simulink library "sm_metronome_lib"  (R2026a)
settings: Solver=VariableStepAuto
undefined symbols (not defined in the file): metronome, X, Y, Z
libraries: sm_lib x11, nesl_utility x3
Description:
  | Copyright 2022-2026 The MathWorks, Inc.
settings Model: Creator=smiller  LastModifiedBy=smiller

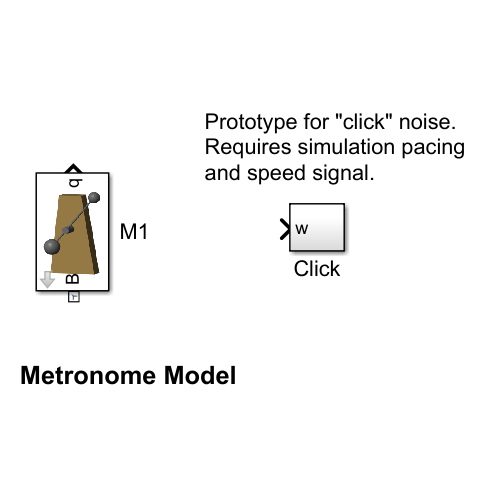
[thumbnail: Simulink's stored preview of the top-level diagram]
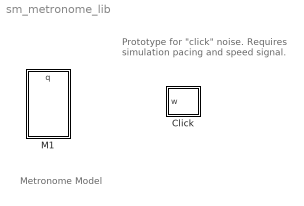
== system sm_metronome_lib ==
  note: Prototype for "click" noise. Requires simulation pacing and speed signal.
  note: Metronome Model
  Click : Subsystem
  M1 : Subsystem  mask(Metronome){pivot_h=metronome.pivot_h, len=metronome.stem_length, upper_len=metronome.stem_upper, upper_len_var=metronome.stem_upper_var, upper_m=metronome.upper_mass, lower_m=metronome.lower_mass, b_pivot=metronome.b_pivot, esc_torque=metronome.esc_torque, t0_ang=metronome.initial_angle(1), t0_vel=metronome.initial_speed(1)}
      mask prompts: pivot_h "Pivot Height (m)"; len "Stem Length (m)"; upper_len "Upper Stem/Length (0-1)"; upper_len_var "Variation in Upper Mass Location (m)"; upper_m "Mass Upper (m)"; lower_m "Mass Lower (m)"; b_pivot "Pivot Viscous Friction (N*m/(deg/s^2))"; esc_torque "Escapement Excitation Torque (N*m)"; t0_ang "Initial Angle (deg)"; t0_vel "Initial Speed (deg/s)"
      mask help: Models a metronome. The pendulum can swing back and forth. Contains abstract model of the energy imparted to the pendulum by the escapement mechanism.
      mask Display: image('sm_metronome_sync_metronome.png');

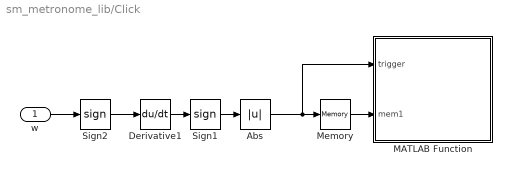
== system sm_metronome_lib/Click ==
  w : Inport
  Abs : Abs  SaturateOnIntegerOverflow=off
  Derivative1 : Derivative
  MATLAB Function : MATLAB Function  TreatAsAtomicUnit=on
  Memory : Memory  InheritSampleTime=on
  Sign1 : Signum
  Sign2 : Signum
  wires:
  Sign2/1 -> Derivative1/1
  Memory/1 -> MATLAB Function/2(mem1)
  w/1 -> Sign2/1
  Sign1/1 -> Abs/1
  Abs/1 -> Memory/1, MATLAB Function/1(trigger)
  Derivative1/1 -> Sign1/1

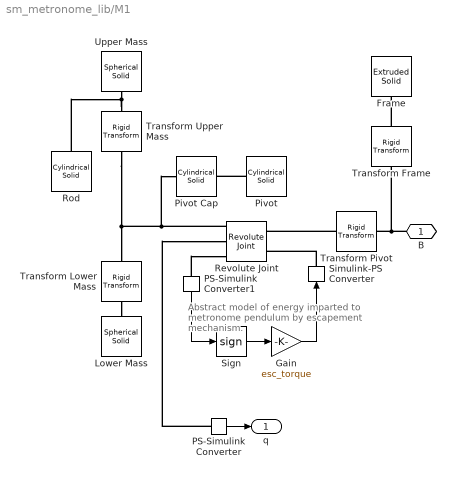
== system sm_metronome_lib/M1 ==
  note: Abstract model of energy imparted
      | to metronome pendulum
      | by escapement mechanism.
  Frame : sm_lib/Body Elements/Extruded Solid  ExtrusionType=General  PolygonNumSides=3  PolygonOuterRadius=1  PolygonOuterRadiusUnits=m  ExportEntireGeometry=off  ExtrusionCrossSection=[4 0; 2 14; -2 14; -4 0]/100  ExtrusionCrossSectionUnits=m  ExportConvexHullGeometry=off  ExtrusionLength=0.02  ExtrusionLengthUnits=m  InertiaType=CalculateFromGeometry  BasedOnType=Mass  Density=1000  DensityUnits=kg/m^3  Mass=0  MassUnits=kg  CenterOfMass=[0 0 0]  CenterOfMassUnits=m  MomentsOfInertia=[1 1 1]  MomentsOfInertiaUnits=kg*m^2  ProductsOfInertia=[0 0 0]  ProductsOfInertiaUnits=kg*m^2  GraphicType=FromGeometry  MarkerShape=Sphere  MarkerSize=10  GraphicVisPropType=SimpleVisualProperties  GraphicDiffuseColor=[0.7372549 0.6039216 0.3372549]  GraphicOpacity=1.0  GraphicSpecularColor=[0.5 0.5 0.5 1.0]  GraphicAmbientColor=[0.15 0.15 0.15 1.0]  GraphicEmissiveColor=[0.0 0.0 0.0 1.0]  GraphicShininess=75  DoExposeReferenceFrame=on  SerializedFrames=<Frames/>
  Gain : Gain  Gain=esc_torque
  Lower Mass : sm_lib/Body Elements/Spherical Solid  SphereRadius=0.014  SphereRadiusUnits=m  ExportEntireGeometry=off  InertiaType=CalculateFromGeometry  BasedOnType=Mass  Density=7600  DensityUnits=kg/m^3  Mass=lower_m  MassUnits=kg  CenterOfMass=[0 0 0]  CenterOfMassUnits=m  MomentsOfInertia=[1 1 1]  MomentsOfInertiaUnits=kg*m^2  ProductsOfInertia=[0 0 0]  ProductsOfInertiaUnits=kg*m^2  GraphicType=FromGeometry  MarkerShape=Sphere  MarkerSize=10  GraphicVisPropType=SimpleVisualProperties  GraphicDiffuseColor=[0.5 0.5 0.5]  GraphicOpacity=1.0  GraphicSpecularColor=[0.5 0.5 0.5 1.0]  GraphicAmbientColor=[0.15 0.15 0.15 1.0]  GraphicEmissiveColor=[0.0 0.0 0.0 1.0]  GraphicShininess=75  DoExposeReferenceFrame=on  SerializedFrames=<Frames/>
  PS-Simulink Converter : nesl_utility/PS-Simulink Converter  PhysicalDomain=network_engine_domain  SubClassName=ps_output  LeftPortType=input  RightPortType=output  PseudoPeriodic=off  Frequencies=[]  VectorFormat=1-D array  Unit=inherit  AffineConversion=off
  PS-Simulink Converter1 : nesl_utility/PS-Simulink Converter  PhysicalDomain=network_engine_domain  SubClassName=ps_output  LeftPortType=input  RightPortType=output  PseudoPeriodic=off  Frequencies=[]  VectorFormat=1-D array  Unit=inherit  AffineConversion=off
  Pivot : sm_lib/Body Elements/Cylindrical Solid  CylinderRadius=len/20  CylinderRadiusUnits=m  CylinderLength=0.03  CylinderLengthUnits=m  ExportEntireGeometry=off  InertiaType=CalculateFromGeometry  BasedOnType=Mass  Density=0  DensityUnits=kg/m^3  Mass=0  MassUnits=kg  CenterOfMass=[0 0 0]  CenterOfMassUnits=m  MomentsOfInertia=[1 1 1]  MomentsOfInertiaUnits=kg*m^2  ProductsOfInertia=[0 0 0]  ProductsOfInertiaUnits=kg*m^2  GraphicType=FromGeometry  MarkerShape=Sphere  MarkerSize=10  GraphicVisPropType=SimpleVisualProperties  GraphicDiffuseColor=[0.5 0.5 0.5]  GraphicOpacity=1.0  GraphicSpecularColor=[0.5 0.5 0.5 1.0]  GraphicAmbientColor=[0.15 0.15 0.15 1.0]  GraphicEmissiveColor=[0.0 0.0 0.0 1.0]  GraphicShininess=75  DoExposeReferenceFrame=off  SerializedFrames=<Frames><Frame><Id>Frame1</Id><Value><Name>Top</Name><Origin><Source>GeometricFeature</Source><FeatureName>top surface</FeatureName></Origin><PrimaryAxis><DefinedDirection>+Z</DefinedDirection><Source>ReferenceFrame</Source><SourceDirection>+Z</SourceDirection><FeatureName></FeatureName></PrimaryAxis><SecondaryAxis><DefinedDirection>+X</DefinedDirection><Source>ReferenceFrame</Source><SourceDirection>+X</SourceDirection><FeatureName></FeatureName></SecondaryAxis></Value></Frame></Frames>
  Pivot Cap : sm_lib/Body Elements/Cylindrical Solid  CylinderRadius=len/20  CylinderRadiusUnits=m  CylinderLength=len/20  CylinderLengthUnits=m  ExportEntireGeometry=off  InertiaType=CalculateFromGeometry  BasedOnType=Mass  Density=0  DensityUnits=kg/m^3  Mass=0  MassUnits=kg  CenterOfMass=[0 0 0]  CenterOfMassUnits=m  MomentsOfInertia=[1 1 1]  MomentsOfInertiaUnits=kg*m^2  ProductsOfInertia=[0 0 0]  ProductsOfInertiaUnits=kg*m^2  GraphicType=FromGeometry  MarkerShape=Sphere  MarkerSize=10  GraphicVisPropType=SimpleVisualProperties  GraphicDiffuseColor=[0.5 0.5 0.5]  GraphicOpacity=1.0  GraphicSpecularColor=[0.5 0.5 0.5 1.0]  GraphicAmbientColor=[0.15 0.15 0.15 1.0]  GraphicEmissiveColor=[0.0 0.0 0.0 1.0]  GraphicShininess=75  DoExposeReferenceFrame=on  SerializedFrames=<Frames><Frame><Id>Frame1</Id><Value><Name>Bot</Name><Origin><Source>GeometricFeature</Source><FeatureName>bottom surface</FeatureName></Origin><PrimaryAxis><DefinedDirection>+Z</DefinedDirection><Source>ReferenceFrame</Source><SourceDirection>+Z</SourceDirection><FeatureName></FeatureName></PrimaryAxis><SecondaryAxis><DefinedDirection>+X</DefinedDirection><Source>ReferenceFrame</Source><SourceDirection>+X</SourceDirection><FeatureName></FeatureName></SecondaryAxis></Value></Frame></Frames>
  Revolute Joint : sm_lib/Joints/Revolute Joint  JointMode=Normal  CompositeWrenchDir=FollowerOnBase  CompositeWrenchFrame=BaseFrame  SenseConstraintForce=off  SenseConstraintTorque=off  SenseTotalForce=off  SenseTotalTorque=off  PositionTargetSpecify=on  PositionTargetPriority=High  PositionTargetValue=t0_ang  PositionTargetValueUnits=deg  VelocityTargetSpecify=on  VelocityTargetPriority=High  VelocityTargetValue=t0_vel  VelocityTargetValueUnits=deg/s  EquilibriumPosition=0  EquilibriumPositionUnits=deg  SpringStiffness=0  SpringStiffnessUnits=N*m/deg  DampingCoefficient=b_pivot  DampingCoefficientUnits=N*m/(deg/s)  LowerLimitSpecify=off  LowerLimitBound=-90  LowerLimitBoundUnits=deg  LowerLimitStiffness=1e4  LowerLimitStiffnessUnits=N*m/deg  LowerLimitDamping=10  LowerLimitDampingUnits=N*m/(deg/s)  LowerLimitTransitionRegionWidth=0.1  LowerLimitTransitionRegionWidthUnits=deg  UpperLimitSpecify=off  UpperLimitBound=90  UpperLimitBoundUnits=deg  UpperLimitStiffness=1e4  UpperLimitStiffnessUnits=N*m/deg  UpperLimitDamping=10  UpperLimitDampingUnits=N*m/(deg/s)  UpperLimitTransitionRegionWidth=0.1  UpperLimitTransitionRegionWidthUnits=deg  TorqueActuationMode=InputTorque  MotionActuationMode=ComputedMotion  SensePosition=on  SenseVelocity=on  SenseAcceleration=off  SenseTorqueForce=off  SenseLowerLimitTorqueForce=off  SenseUpperLimitTorqueForce=off
  Rod : sm_lib/Body Elements/Cylindrical Solid  CylinderRadius=len/80  CylinderRadiusUnits=m  CylinderLength=len  CylinderLengthUnits=m  ExportEntireGeometry=off  InertiaType=CalculateFromGeometry  BasedOnType=Mass  Density=1000  DensityUnits=kg/m^3  Mass=0  MassUnits=kg  CenterOfMass=[0 0 0]  CenterOfMassUnits=m  MomentsOfInertia=[1 1 1]  MomentsOfInertiaUnits=kg*m^2  ProductsOfInertia=[0 0 0]  ProductsOfInertiaUnits=kg*m^2  GraphicType=FromGeometry  MarkerShape=Sphere  MarkerSize=10  GraphicVisPropType=SimpleVisualProperties  GraphicDiffuseColor=[0.5 0.5 0.5]  GraphicOpacity=1.0  GraphicSpecularColor=[0.5 0.5 0.5 1.0]  GraphicAmbientColor=[0.15 0.15 0.15 1.0]  GraphicEmissiveColor=[0.0 0.0 0.0 1.0]  GraphicShininess=75  DoExposeReferenceFrame=off  SerializedFrames=<Frames><Frame><Id>Frame1</Id><Value><Name>Top</Name><Origin><Source>GeometricFeature</Source><FeatureName>top surface</FeatureName></Origin><PrimaryAxis><DefinedDirection>+Z</DefinedDirection><Source>ReferenceFrame</Source><SourceDirection>-Y</SourceDirection><FeatureName></FeatureName></PrimaryAxis><SecondaryAxis><DefinedDirection>+X</DefinedDirection><Source>ReferenceFrame</Source><SourceDirection>+X</SourceDirection><FeatureName></FeatureName></SecondaryAxis></Value></Frame></Frames>
  Sign : Signum  ZeroCross=off
  Simulink-PS Converter : nesl_utility/Simulink-PS Converter  PhysicalDomain=network_engine_domain  SubClassName=ps_input  LeftPortType=input  RightPortType=output  PseudoPeriodic=off  Frequencies=[]  NoiseDistribution=none  NoiseParameters=[]  Unit=1  AffineConversion=off  FilteringAndDerivatives=provide  SimscapeFilterOrder=1  InputFilterTimeConstant=0.001  UdotUserProvided=0
  Transform Frame : sm_lib/Frames and Transforms/Rigid Transform  RotationMethod=StandardAxis  FollAlignAxisA=+X  BaseAlignAxisA=+Y  FollAlignAxisB=+Y  BaseAlignAxisB=+Z  RotationStandardAxis=+X  RotationAngle=90  RotationAngleUnits=deg  RotationArbitraryAxis=[0 0 1]  RotationSequenceAxes=FollowerAxes  RotationSequence=XYX  RotationSequenceAngles=[0 0 0]  RotationSequenceAnglesUnits=deg  RotationMatrix=[1 0 0; 0 1 0; 0 0 1]  Quaternion=[1 0 0 0]  TranslationMethod=StandardAxis  TranslationCartesianOffset=[0 0 0]  TranslationCartesianOffsetUnits=m  TranslationStandardAxis=+Y  TranslationStandardOffset=0.03  TranslationStandardOffsetUnits=m  TranslationROffset=0  TranslationROffsetUnits=m  TranslationThetaOffset=0  TranslationThetaOffsetUnits=deg  TranslationZOffset=0  TranslationZOffsetUnits=m
  Transform Lower Mass : sm_lib/Frames and Transforms/Rigid Transform  RotationMethod=None  FollAlignAxisA=+X  BaseAlignAxisA=+Y  FollAlignAxisB=+Y  BaseAlignAxisB=+Z  RotationStandardAxis=+Z  RotationAngle=0.0  RotationAngleUnits=deg  RotationArbitraryAxis=[0 0 1]  RotationSequenceAxes=FollowerAxes  RotationSequence=XYX  RotationSequenceAngles=[0 0 0]  RotationSequenceAnglesUnits=deg  RotationMatrix=[1 0 0; 0 1 0; 0 0 1]  Quaternion=[1 0 0 0]  TranslationMethod=StandardAxis  TranslationCartesianOffset=[0 -0.04 0]  TranslationCartesianOffsetUnits=m  TranslationStandardAxis=+Y  TranslationStandardOffset=-len*(1-upper_len)  TranslationStandardOffsetUnits=m  TranslationROffset=0  TranslationROffsetUnits=m  TranslationThetaOffset=0  TranslationThetaOffsetUnits=deg  TranslationZOffset=0  TranslationZOffsetUnits=m
  Transform Pivot : sm_lib/Frames and Transforms/Rigid Transform  RotationMethod=StandardAxis  FollAlignAxisA=+X  BaseAlignAxisA=+Y  FollAlignAxisB=+Y  BaseAlignAxisB=+Z  RotationStandardAxis=+X  RotationAngle=90  RotationAngleUnits=deg  RotationArbitraryAxis=[0 0 1]  RotationSequenceAxes=FollowerAxes  RotationSequence=XYX  RotationSequenceAngles=[0 0 0]  RotationSequenceAnglesUnits=deg  RotationMatrix=[1 0 0; 0 1 0; 0 0 1]  Quaternion=[1 0 0 0]  TranslationMethod=StandardAxis  TranslationCartesianOffset=[0 0 0]  TranslationCartesianOffsetUnits=m  TranslationStandardAxis=+Z  TranslationStandardOffset=pivot_h  TranslationStandardOffsetUnits=m  TranslationROffset=0  TranslationROffsetUnits=m  TranslationThetaOffset=0  TranslationThetaOffsetUnits=deg  TranslationZOffset=0  TranslationZOffsetUnits=m
  Transform Upper Mass : sm_lib/Frames and Transforms/Rigid Transform  RotationMethod=None  FollAlignAxisA=+X  BaseAlignAxisA=+Y  FollAlignAxisB=+Y  BaseAlignAxisB=+Z  RotationStandardAxis=+Z  RotationAngle=0.0  RotationAngleUnits=deg  RotationArbitraryAxis=[0 0 1]  RotationSequenceAxes=FollowerAxes  RotationSequence=XYX  RotationSequenceAngles=[0 0 0]  RotationSequenceAnglesUnits=deg  RotationMatrix=[1 0 0; 0 1 0; 0 0 1]  Quaternion=[1 0 0 0]  TranslationMethod=StandardAxis  TranslationCartesianOffset=[0 0.08 0]  TranslationCartesianOffsetUnits=m  TranslationStandardAxis=+Y  TranslationStandardOffset=len*upper_len+upper_len_var*(-1+2*rand(1,1))  TranslationStandardOffsetUnits=m  TranslationROffset=0  TranslationROffsetUnits=m  TranslationThetaOffset=0  TranslationThetaOffsetUnits=deg  TranslationZOffset=0  TranslationZOffsetUnits=m
  Upper Mass : sm_lib/Body Elements/Spherical Solid  SphereRadius=0.01  SphereRadiusUnits=m  ExportEntireGeometry=off  InertiaType=CalculateFromGeometry  BasedOnType=Mass  Density=7600  DensityUnits=kg/m^3  Mass=upper_m  MassUnits=kg  CenterOfMass=[0 0 0]  CenterOfMassUnits=m  MomentsOfInertia=[1 1 1]  MomentsOfInertiaUnits=kg*m^2  ProductsOfInertia=[0 0 0]  ProductsOfInertiaUnits=kg*m^2  GraphicType=FromGeometry  MarkerShape=Sphere  MarkerSize=10  GraphicVisPropType=SimpleVisualProperties  GraphicDiffuseColor=[0.5 0.5 0.5]  GraphicOpacity=1.0  GraphicSpecularColor=[0.5 0.5 0.5 1.0]  GraphicAmbientColor=[0.15 0.15 0.15 1.0]  GraphicEmissiveColor=[0.0 0.0 0.0 1.0]  GraphicShininess=75  DoExposeReferenceFrame=on  SerializedFrames=<Frames/>
  B : PMIOPort  Side=Left
  q : Outport
  wires:
  PS-Simulink Converter/1 -> q/1
  Gain/1 -> Simulink-PS Converter/1
  Sign/1 -> Gain/1
  PS-Simulink Converter1/1 -> Sign/1
  connections:
  PS-Simulink Converter/LConn1 -- Revolute Joint/RConn2
  Upper Mass/RConn1 -- Rod/LConn1 -- Transform Upper Mass/RConn1
  Transform Pivot/LConn1 -- B/RConn1 -- Transform Frame/LConn1
  Transform Upper Mass/LConn1 -- Revolute Joint/RConn1 -- Pivot Cap/RConn1 -- Transform Lower Mass/LConn1
  Transform Lower Mass/RConn1 -- Lower Mass/RConn1
  Transform Pivot/RConn1 -- Revolute Joint/LConn1
  PS-Simulink Converter1/LConn1 -- Revolute Joint/RConn3
  Simulink-PS Converter/RConn1 -- Revolute Joint/LConn2
  Transform Frame/RConn1 -- Frame/RConn1
  Pivot/LConn1 -- Pivot Cap/LConn1

== matlab function sm_metronome_lib/Click/MATLAB Function ==
  data: trigger input; mem1 input
function fcn(trigger,mem1)
coder.extrinsic('sound');
if trigger == 1 && mem1 ~= 1

Fs = 44100;
b = [0.0109252929687500;0.0116882324218750;0.0122680664062500;0.0130615234375000;0.0144348144531250;0.0161743164062500;0.0177307128906250;0.0198669433593750;0.0233459472656250;0.0292358398437500;0.0350646972656250;0.0434570312500000;0.0539245605468750;0.0662536621093750;0.0837402343750000;0.105804443359375;0.126007080078125;0.142578125000000;0.150939941406250;0.155456542968750;0.155273437500000;0.135131835937500;0.106933593750000;0.0668334960937500;-0.00140380859375000;-0.0640258789062500;-0.0463562011718750;-0.0270690917968750;-0.0557556152343750;-0.0654296875000000;-0.0552978515625000;-0.0486755371093750;-0.0500793457031250;-0.0796508789062500;-0.0970458984375000;-0.0562744140625000;-0.0451354980468750;-0.105194091796875;-0.173553466796875;-0.178070068359375;-0.206237792968750;-0.268402099609375;-0.251281738281250;-0.150329589843750;-0.0434265136718750;0.0223693847656250;0.0999145507812500;0.138092041015625;0.0578308105468750;-0.0370178222656250;-0.0488891601562500;0.00115966796875000;0.0530090332031250;0.0529785156250000;0.0611877441406250;0.0783081054687500;0.0502014160156250;0.0245971679687500;0.0184631347656250;0.0228271484375000;0.0278625488281250;0.0287780761718750;0.0303955078125000;0.0151672363281250;-0.00173950195312500;-0.0346679687500000;-0.0734558105468750;-0.114501953125000;-0.160888671875000;-0.186798095703125;-0.176452636718750;-0.103607177734375;-0.0356445312500000;-0.0120544433593750;0.00756835937500000;0.00741577148437500;-0.0498352050781250;-0.134582519531250;-0.218933105468750;-0.255737304687500;-0.218566894531250;-0.133789062500000;-0.0301513671875000;0.0305786132812500;0.0281982421875000;-0.0208435058593750;-0.106506347656250;-0.175750732421875;-0.162841796875000;-0.104187011718750;-0.0490417480468750;-0.00372314453125000;0.0379638671875000;0.0422973632812500;0.0299987792968750;0.0311279296875000;0.0163269042968750;0.000640869140625000;0.0194702148437500;0.0485229492187500;0.0509948730468750;0.0360412597656250;0.0467834472656250;0.0584716796875000;0.0416564941406250;0.0204467773437500;0.0122985839843750;-0.00408935546875000;-0.0237426757812500;-0.0214538574218750;-0.00546264648437500;0.00216674804687500;0.00836181640625000;0.00698852539062500;-0.0217895507812500;-0.0512695312500000;-0.0408630371093750;-0.0181274414062500;-0.0165710449218750;-0.00720214843750000;0.00802612304687500;-0.0101623535156250;-0.0533447265625000;-0.0711364746093750;-0.0697326660156250;-0.0811767578125000;-0.0798950195312500;-0.0582275390625000;-0.0451965332031250;-0.0513916015625000;-0.0266723632812500;0.0344848632812500;0.0915527343750000;0.125640869140625;0.135894775390625;0.117706298828125;0.0757446289062500;0.0403137207031250;0.0227966308593750;0.00469970703125000;-0.0107116699218750;-0.0209960937500000;-0.0346984863281250;-0.0541992187500000;-0.0585937500000000;-0.0434265136718750;-0.0420837402343750;-0.0512390136718750;-0.0430297851562500;-0.0332946777343750;-0.0376586914062500;-0.0476684570312500;-0.0518188476562500;-0.0502319335937500;-0.0403137207031250;-0.0241394042968750;0.00152587890625000;0.0372314453125000;0.0740051269531250;0.0895996093750000;0.0790710449218750;0.0711059570312500;0.0841674804687500;0.106109619140625;0.119628906250000;0.131072998046875;0.130310058593750;0.107543945312500;0.0800476074218750;0.0597534179687500;0.0526428222656250;0.0576477050781250;0.0683288574218750;0.0789184570312500;0.0751647949218750;0.0584106445312500;0.0457763671875000;0.0424804687500000;0.0377502441406250;0.0230407714843750;0.00430297851562500;-0.00857543945312500;-0.0210571289062500;-0.0342712402343750;-0.0408935546875000;-0.0378417968750000;-0.0221862792968750;0.00857543945312500;0.0375671386718750;0.0588684082031250;0.0796508789062500;0.106719970703125;0.129180908203125;0.144134521484375;0.160064697265625;0.166351318359375;0.152709960937500;0.133666992187500;0.114501953125000;0.0937194824218750;0.0732421875000000;0.0662231445312500;0.0630798339843750;0.0375976562500000;0.00958251953125000;-0.0138854980468750;-0.0361938476562500;-0.0600280761718750;-0.0831909179687500;-0.0963745117187500;-0.110443115234375;-0.119750976562500;-0.118621826171875;-0.115722656250000;-0.105163574218750;-0.0841064453125000;-0.0640869140625000;-0.0502929687500000;-0.0397338867187500;-0.0249328613281250;-0.00503540039062500;0.0149841308593750;0.0276794433593750;0.0352478027343750;0.0420837402343750;0.0440063476562500;0.0483093261718750;0.0517883300781250;0.0487365722656250;0.0476989746093750;0.0537719726562500;0.0480651855468750;0.0399169921875000;0.0335388183593750;0.0180664062500000;-0.000579833984375000;-0.00735473632812500;0.0106811523437500;0.0154113769531250;-0.00134277343750000;-0.00192260742187500;0.0124511718750000;0.0282287597656250;0.0362243652343750;0.0399780273437500;0.0453491210937500;0.0490722656250000;0.0598144531250000;0.0744323730468750;0.0884094238281250;0.0975952148437500;0.0921020507812500;0.0725097656250000;0.0568542480468750;0.0535278320312500;0.0600280761718750;0.0776977539062500;0.0849304199218750;0.0697631835937500;0.0578308105468750;0.0520324707031250;0.0395202636718750;0.0247192382812500;0.0157775878906250;0.0136108398437500;0.0171508789062500;0.0151977539062500;0.00680541992187500;-0.00549316406250000;-0.0202026367187500;-0.0321655273437500;-0.0405273437500000;-0.0521545410156250;-0.0687866210937500;-0.0847167968750000;-0.0952758789062500;-0.0919494628906250;-0.0808105468750000;-0.0732116699218750;-0.0664367675781250;-0.0654602050781250;-0.0635070800781250;-0.0523681640625000;-0.0358581542968750;-0.0197143554687500;-0.0118713378906250;-0.0144348144531250;-0.0188598632812500;-0.0251159667968750;-0.0309753417968750;-0.0342407226562500;-0.0329284667968750;-0.0292053222656250;-0.0235595703125000;-0.0183105468750000;-0.0152282714843750;-0.0140075683593750;-0.0161437988281250;-0.0223999023437500;-0.0327453613281250;-0.0391235351562500;-0.0455627441406250;-0.0527954101562500;-0.0543518066406250;-0.0508422851562500;-0.0463867187500000;-0.0457763671875000;-0.0428466796875000;-0.0410766601562500;-0.0409240722656250;-0.0372314453125000;-0.0309143066406250;-0.0208740234375000;-0.00912475585937500;-0.00216674804687500;-0.00485229492187500;-0.0162048339843750;-0.0293884277343750;-0.0366210937500000;-0.0381774902343750;-0.0362548828125000;-0.0344238281250000;-0.0327453613281250;-0.0273132324218750;-0.0227966308593750;-0.0280456542968750;-0.0367736816406250;-0.0395812988281250;-0.0387573242187500;-0.0364074707031250;-0.0358276367187500;-0.0424499511718750;-0.0483398437500000;-0.0463867187500000;-0.0447998046875000;-0.0469055175781250;-0.0467529296875000;-0.0438232421875000;-0.0407104492187500;-0.0343017578125000;-0.0219726562500000;-0.0119018554687500;-0.00521850585937500;0.00189208984375000;0.00759887695312500;0.0116882324218750;0.0136718750000000;0.0165405273437500;0.0235595703125000;0.0290222167968750;0.0313415527343750;0.0317687988281250;0.0340881347656250;0.0401000976562500;0.0444335937500000;0.0461730957031250;0.0463562011718750;0.0479125976562500;0.0494995117187500;0.0459594726562500;0.0364379882812500;0.0270690917968750;0.0173339843750000;0.00390625000000000;-0.00897216796875000;-0.0159301757812500;-0.0218505859375000;-0.0305786132812500;-0.0340881347656250;-0.0305175781250000;-0.0255737304687500;-0.0245361328125000;-0.0288085937500000;-0.0339355468750000;-0.0373840332031250;-0.0397338867187500;-0.0379638671875000;-0.0311584472656250;-0.0257568359375000;-0.0249328613281250;-0.0255126953125000;-0.0257263183593750;-0.0280456542968750;-0.0319519042968750;-0.0348205566406250;-0.0321655273437500;-0.0285949707031250;-0.0274963378906250;-0.0261230468750000;-0.0256652832031250;-0.0280456542968750;-0.0317687988281250;-0.0372009277343750;-0.0421142578125000;-0.0436096191406250;-0.0416870117187500;-0.0397338867187500;-0.0364074707031250;-0.0364074707031250;-0.0407104492187500;-0.0455932617187500;-0.0516052246093750;-0.0578918457031250;-0.0607604980468750;-0.0635375976562500;-0.0640563964843750;-0.0594482421875000;-0.0549011230468750;-0.0521850585937500;-0.0459594726562500;-0.0366210937500000;-0.0303955078125000;-0.0252990722656250;-0.0179138183593750;-0.00646972656250000;0.00408935546875000;0.0126647949218750;0.0212707519531250;0.0270385742187500;0.0294494628906250;0.0285949707031250;0.0272827148437500;0.0274658203125000;0.0262756347656250;0.0255126953125000;0.0282287597656250;0.0303955078125000;0.0296325683593750;0.0285949707031250;0.0276794433593750;0.0267028808593750;0.0276184082031250;0.0323486328125000;0.0399475097656250;0.0471496582031250;0.0537414550781250;0.0563049316406250;0.0567016601562500;0.0609436035156250;0.0668029785156250;0.0707397460937500;0.0751953125000000;0.0825500488281250;0.0903930664062500;0.0954589843750000;0.0981750488281250;0.0977783203125000;0.0961914062500000;0.0948791503906250;0.0936889648437500;0.0931091308593750;0.0935058593750000;0.0907287597656250;0.0855407714843750;0.0811767578125000;0.0765991210937500;0.0690917968750000;0.0596618652343750;0.0486755371093750;0.0393371582031250;0.0297851562500000;0.0220336914062500;0.0159606933593750;0.00915527343750000;0.00198364257812500;-0.00531005859375000;-0.0104980468750000;-0.0151977539062500;-0.0204162597656250;-0.0249633789062500;-0.0264587402343750;-0.0280151367187500;-0.0300292968750000;-0.0303344726562500;-0.0311584472656250;-0.0319519042968750;-0.0315551757812500;-0.0317687988281250;-0.0317382812500000;-0.0321655273437500;-0.0327148437500000;-0.0327453613281250;-0.0336914062500000;-0.0350036621093750;-0.0362243652343750;-0.0381774902343750;-0.0432739257812500;-0.0488891601562500;-0.0546875000000000;-0.0596618652343750;-0.0613098144531250;-0.0621643066406250;-0.0617370605468750;-0.0603637695312500;-0.0592041015625000;-0.0578308105468750;-0.0569152832031250;-0.0537414550781250;-0.0467529296875000;-0.0389404296875000;-0.0298156738281250;-0.0204162597656250;-0.0134277343750000;-0.00704956054687500;0.000579833984375000;0.00723266601562500;0.0113220214843750;0.0151977539062500;0.0169067382812500;0.0171508789062500;0.0158081054687500;0.0151672363281250;0.0153808593750000;0.0136413574218750;0.0103454589843750;0.00738525390625000;0.00561523437500000;0.00369262695312500;0.00198364257812500;0.00119018554687500;0.00231933593750000;0.00314331054687500;0.00170898437500000;0.000396728515625000;0.000183105468750000;-0.000183105468750000;0.000213623046875000;0.000366210937500000;0.000183105468750000;0.000610351562500000;0.00155639648437500;0.00238037109375000;0.00347900390625000;0.00570678710937500;0.00872802734375000;0.0101318359375000;0.0103454589843750;0.00991821289062500;0.00939941406250000;0.00933837890625000;0.0104980468750000;0.0122375488281250;0.0134277343750000;0.0134582519531250;0.0144348144531250;0.0153808593750000;0.0150146484375000;0.0151367187500000;0.0171813964843750;0.0179443359375000;0.0186767578125000;0.0198974609375000;0.0211791992187500;0.0226135253906250;0.0227661132812500;0.0222778320312500;0.0210266113281250;0.0184631347656250;0.0152282714843750;0.0118713378906250;0.00894165039062500;0.00546264648437500;0.00231933593750000;0.000183105468750000;-0.00192260742187500;-0.00524902343750000;-0.00915527343750000;-0.0109252929687500;-0.0115051269531250;-0.0132141113281250;-0.0138549804687500;-0.0128784179687500;-0.0134277343750000;-0.0157775878906250;-0.0184936523437500;-0.0212402343750000;-0.0227355957031250;-0.0235900878906250;-0.0249023437500000;-0.0270996093750000;-0.0302124023437500;-0.0325317382812500;-0.0333251953125000;-0.0352478027343750;-0.0356445312500000;-0.0371704101562500;-0.0379638671875000;-0.0383911132812500;-0.0399475097656250;-0.0411071777343750;-0.0408935546875000;-0.0383911132812500;-0.0375671386718750;-0.0381774902343750;-0.0399780273437500;-0.0412902832031250;-0.0417175292968750;-0.0422363281250000;-0.0420837402343750;-0.0412597656250000;-0.0407409667968750;-0.0401000976562500;-0.0393676757812500;-0.0383300781250000;-0.0366210937500000;-0.0341186523437500;-0.0311584472656250;-0.0284423828125000;-0.0251464843750000;-0.0223388671875000;-0.0202941894531250;-0.0179138183593750;-0.0142517089843750;-0.00955200195312500;-0.00561523437500000;-0.00350952148437500;-0.00234985351562500;-0.000183105468750000;0.00213623046875000;0.00524902343750000;0.00875854492187500;0.0107421875000000;0.0119018554687500;0.0132446289062500;0.0148010253906250;0.0177307128906250;0.0204467773437500;0.0212402343750000;0.0212402343750000;0.0216369628906250;0.0229492187500000;0.0239562988281250;0.0245971679687500;0.0243530273437500;0.0231628417968750;0.0223999023437500;0.0212707519531250;0.0200500488281250;0.0187072753906250;0.0178833007812500;0.0184936523437500;0.0206298828125000;0.0233764648437500;0.0263366699218750;0.0283813476562500;0.0309753417968750;0.0333251953125000;0.0328979492187500;0.0331420898437500;0.0340881347656250;0.0352478027343750;0.0358276367187500;0.0354614257812500;0.0348510742187500;0.0348815917968750;0.0334777832031250;0.0303955078125000;0.0266723632812500;0.0241699218750000;0.0210266113281250;0.0169677734375000];
a = [0.00784301757812500;0.00717163085937500;0.00701904296875000;0.00643920898437500;0.00604248046875000;0.00622558593750000;0.00622558593750000;0.00662231445312500;0.00662231445312500;0.00857543945312500;0.0128479003906250;0.0173339843750000;0.0258789062500000;0.0393371582031250;0.0572509765625000;0.0857238769531250;0.123687744140625;0.163787841796875;0.196350097656250;0.212341308593750;0.235443115234375;0.243713378906250;0.232147216796875;0.207427978515625;0.147247314453125;0.0337219238281250;-0.0344848632812500;0.0122680664062500;0.0574035644531250;0.0611572265625000;0.0876770019531250;0.0896301269531250;-0.00415039062500000;-0.109069824218750;-0.178436279296875;-0.165924072265625;-0.157379150390625;-0.215026855468750;-0.265716552734375;-0.306182861328125;-0.381927490234375;-0.533905029296875;-0.543273925781250;-0.388153076171875;-0.246643066406250;-0.193389892578125;-0.108703613281250;-0.0652160644531250;-0.127014160156250;-0.189727783203125;-0.122924804687500;-0.0418395996093750;-0.0228271484375000;-0.0276184082031250;-0.0621948242187500;-0.0711059570312500;-0.0358276367187500;0.0218200683593750;0.0776977539062500;0.145141601562500;0.159118652343750;0.0874633789062500;-0.00213623046875000;-0.0325012207031250;-0.0134582519531250;-0.00680541992187500;0.00271606445312500;-0.000579833984375000;-0.0483398437500000;-0.131805419921875;-0.171997070312500;-0.107543945312500;-0.00622558593750000;0.0557250976562500;0.0669860839843750;0.0714721679687500;0.0188293457031250;-0.0468750000000000;-0.0843505859375000;-0.128784179687500;-0.124481201171875;-0.0814208984375000;-0.0342712402343750;0.0144042968750000;0.0389709472656250;0.0237731933593750;-0.0222167968750000;-0.0432434082031250;-0.00463867187500000;0.0241088867187500;0.0163574218750000;0.0434265136718750;0.0909729003906250;0.107360839843750;0.120147705078125;0.138336181640625;0.131652832031250;0.116851806640625;0.112030029296875;0.120941162109375;0.124084472656250;0.0910949707031250;0.0843811035156250;0.108703613281250;0.0842895507812500;0.0635375976562500;0.0720825195312500;0.0535583496093750;0.0208435058593750;0.0112915039062500;0.0204162597656250;0.0140686035156250;0.00991821289062500;0.0249328613281250;-0.00680541992187500;-0.0383911132812500;-0.0204162597656250;-0.0220642089843750;-0.0592041015625000;-0.0710754394531250;-0.0603637695312500;-0.0734558105468750;-0.0909423828125000;-0.0715026855468750;-0.0615234375000000;-0.0724792480468750;-0.0675659179687500;-0.0446472167968750;-0.0410766601562500;-0.0506591796875000;-0.0255432128906250;0.0327453613281250;0.0820007324218750;0.116302490234375;0.145050048828125;0.146667480468750;0.111267089843750;0.0928955078125000;0.0931091308593750;0.0814514160156250;0.0662231445312500;0.0463256835937500;0.0239562988281250;0.000610351562500000;0.00234985351562500;0.0281982421875000;0.0350646972656250;0.0393981933593750;0.0436096191406250;0.0264892578125000;-0.0107116699218750;-0.0364379882812500;-0.0434265136718750;-0.0350341796875000;-0.00564575195312500;0.0368347167968750;0.0636901855468750;0.102844238281250;0.142578125000000;0.137878417968750;0.106903076171875;0.0989685058593750;0.120971679687500;0.141021728515625;0.149597167968750;0.148590087890625;0.135955810546875;0.109466552734375;0.0742492675781250;0.0537414550781250;0.0465698242187500;0.0483398437500000;0.0636596679687500;0.0776977539062500;0.0680236816406250;0.0418395996093750;0.0278930664062500;0.0194702148437500;0.00195312500000000;-0.0304260253906250;-0.0683593750000000;-0.0940856933593750;-0.108886718750000;-0.116302490234375;-0.108642578125000;-0.0938720703125000;-0.0693969726562500;-0.0350646972656250;-0.00759887695312500;0.00451660156250000;0.0178833007812500;0.0432434082031250;0.0695495605468750;0.0962219238281250;0.121765136718750;0.139221191406250;0.145538330078125;0.134399414062500;0.111419677734375;0.0767517089843750;0.0469055175781250;0.0407714843750000;0.0379333496093750;0.0264892578125000;0.00820922851562500;-0.00778198242187500;-0.0247802734375000;-0.0482788085937500;-0.0711059570312500;-0.0941162109375000;-0.112365722656250;-0.115875244140625;-0.110626220703125;-0.106170654296875;-0.0928955078125000;-0.0722961425781250;-0.0593872070312500;-0.0533752441406250;-0.0502929687500000;-0.0438537597656250;-0.0329284667968750;-0.0161437988281250;0.0108947753906250;0.0399169921875000;0.0586547851562500;0.0683593750000000;0.0798339843750000;0.0814208984375000;0.0713195800781250;0.0661926269531250;0.0693664550781250;0.0673828125000000;0.0691528320312500;0.0724487304687500;0.0563049316406250;0.0268554687500000;0.0206298828125000;0.0164184570312500;-0.00216674804687500;-0.0184936523437500;-0.0216064453125000;-0.00665283203125000;0.0115356445312500;0.0184936523437500;0.0148315429687500;0.0148315429687500;0.0134277343750000;0.0151367187500000;0.0185546875000000;0.0301818847656250;0.0409240722656250;0.0364379882812500;0.0285949707031250;0.0163879394531250;0.00720214843750000;0.0159912109375000;0.0280456542968750;0.0206298828125000;0.0122985839843750;0.00820922851562500;0.00463867187500000;0.00198364257812500;-0.00375366210937500;-0.00564575195312500;-0.00857543945312500;-0.00564575195312500;-0.0106506347656250;-0.0270996093750000;-0.0362243652343750;-0.0502624511718750;-0.0588073730468750;-0.0588073730468750;-0.0631103515625000;-0.0835876464843750;-0.105377197265625;-0.112182617187500;-0.109069824218750;-0.109039306640625;-0.110473632812500;-0.109863281250000;-0.110229492187500;-0.111053466796875;-0.103973388671875;-0.0892333984375000;-0.0787048339843750;-0.0750122070312500;-0.0759277343750000;-0.0763549804687500;-0.0754089355468750;-0.0751953125000000;-0.0720214843750000;-0.0652770996093750;-0.0594177246093750;-0.0529479980468750;-0.0444335937500000;-0.0385437011718750;-0.0344848632812500;-0.0334777832031250;-0.0395507812500000;-0.0523986816406250;-0.0582580566406250;-0.0658264160156250;-0.0775451660156250;-0.0825805664062500;-0.0864868164062500;-0.0870666503906250;-0.0868835449218750;-0.0897827148437500;-0.0884704589843750;-0.0858459472656250;-0.0822143554687500;-0.0740051269531250;-0.0596313476562500;-0.0455627441406250;-0.0352478027343750;-0.0335083007812500;-0.0407104492187500;-0.0479125976562500;-0.0506591796875000;-0.0469665527343750;-0.0433959960937500;-0.0442199707031250;-0.0432434082031250;-0.0387878417968750;-0.0345153808593750;-0.0340881347656250;-0.0352478027343750;-0.0334777832031250;-0.0325317382812500;-0.0288391113281250;-0.0299682617187500;-0.0403747558593750;-0.0457763671875000;-0.0431823730468750;-0.0395812988281250;-0.0397338867187500;-0.0426635742187500;-0.0436401367187500;-0.0416870117187500;-0.0340576171875000;-0.0200500488281250;-0.0107421875000000;-0.00253295898437500;0.00549316406250000;0.00970458984375000;0.0138549804687500;0.0179138183593750;0.0237731933593750;0.0323181152343750;0.0372314453125000;0.0375366210937500;0.0368347167968750;0.0395202636718750;0.0414733886718750;0.0422668457031250;0.0415039062500000;0.0364074707031250;0.0331420898437500;0.0261230468750000;0.0147705078125000;0.00524902343750000;-0.00500488281250000;-0.0181274414062500;-0.0350952148437500;-0.0477294921875000;-0.0552978515625000;-0.0648193359375000;-0.0724792480468750;-0.0755920410156250;-0.0715332031250000;-0.0634460449218750;-0.0611877441406250;-0.0644836425781250;-0.0675964355468750;-0.0720825195312500;-0.0763549804687500;-0.0730285644531250;-0.0678100585937500;-0.0664062500000000;-0.0652465820312500;-0.0632934570312500;-0.0596313476562500;-0.0605468750000000;-0.0619812011718750;-0.0584106445312500;-0.0560913085937500;-0.0535583496093750;-0.0502929687500000;-0.0465393066406250;-0.0432434082031250;-0.0395507812500000;-0.0383605957031250;-0.0383911132812500;-0.0383300781250000;-0.0343017578125000;-0.0274353027343750;-0.0247802734375000;-0.0227661132812500;-0.0233764648437500;-0.0276489257812500;-0.0321350097656250;-0.0358276367187500;-0.0389709472656250;-0.0404968261718750;-0.0415039062500000;-0.0422668457031250;-0.0397033691406250;-0.0368652343750000;-0.0344848632812500;-0.0249328613281250;-0.0134277343750000;-0.00625610351562500;0.00238037109375000;0.0140075683593750;0.0280456542968750;0.0418701171875000;0.0534362792968750;0.0642700195312500;0.0730285644531250;0.0763854980468750;0.0749816894531250;0.0732421875000000;0.0716552734375000;0.0687561035156250;0.0691528320312500;0.0724792480468750;0.0745544433593750;0.0750427246093750;0.0755310058593750;0.0750427246093750;0.0759277343750000;0.0787048339843750;0.0827941894531250;0.0907897949218750;0.0999145507812500;0.107330322265625;0.111358642578125;0.115722656250000;0.122344970703125;0.127960205078125;0.128936767578125;0.130737304687500;0.135375976562500;0.139068603515625;0.140411376953125;0.138885498046875;0.136932373046875;0.136566162109375;0.133178710937500;0.129760742187500;0.128387451171875;0.128173828125000;0.123870849609375;0.117645263671875;0.114562988281250;0.111419677734375;0.106353759765625;0.0989074707031250;0.0911865234375000;0.0829467773437500;0.0746154785156250;0.0687561035156250;0.0628967285156250;0.0561218261718750;0.0473022460937500;0.0379943847656250;0.0301818847656250;0.0237731933593750;0.0171508789062500;0.0109252929687500;0.00659179687500000;0.00271606445312500;-0.000335693359375000;-0.00231933593750000;-0.00646972656250000;-0.00778198242187500;-0.00738525390625000;-0.00622558593750000;-0.00503540039062500;-0.00469970703125000;-0.00390625000000000;-0.00354003906250000;-0.00540161132812500;-0.00741577148437500;-0.00720214843750000;-0.00955200195312500;-0.0138549804687500;-0.0190429687500000;-0.0247497558593750;-0.0303649902343750;-0.0341186523437500;-0.0340270996093750;-0.0354614257812500;-0.0362243652343750;-0.0364379882812500;-0.0379943847656250;-0.0385742187500000;-0.0364074707031250;-0.0334777832031250;-0.0302124023437500;-0.0255432128906250;-0.0208129882812500;-0.0179138183593750;-0.0146179199218750;-0.0104980468750000;-0.00585937500000000;-0.000976562500000000;0.00274658203125000;0.00585937500000000;0.00659179687500000;0.00567626953125000;0.00701904296875000;0.00701904296875000;0.00524902343750000;0.00347900390625000;0.00354003906250000;0.00430297851562500;0.00390625000000000;0.00366210937500000;0.00390625000000000;0.00463867187500000;0.00494384765625000;0.00408935546875000;0.00384521484375000;0.00531005859375000;0.00643920898437500;0.00756835937500000;0.00720214843750000;0.00582885742187500;0.00546264648437500;0.00564575195312500;0.00506591796875000;0.00659179687500000;0.00955200195312500;0.0124816894531250;0.0144348144531250;0.0157775878906250;0.0169067382812500;0.0175781250000000;0.0186767578125000;0.0231628417968750;0.0265197753906250;0.0284118652343750;0.0298461914062500;0.0311584472656250;0.0332946777343750;0.0346069335937500;0.0364685058593750;0.0383605957031250;0.0401611328125000;0.0406494140625000;0.0415344238281250;0.0429992675781250;0.0446472167968750;0.0449523925781250;0.0432434082031250;0.0407104492187500;0.0378112792968750;0.0327453613281250;0.0280456542968750;0.0231628417968750;0.0183105468750000;0.0134277343750000;0.00955200195312500;0.00524902343750000;-0.000427246093750000;-0.00500488281250000;-0.00704956054687500;-0.00933837890625000;-0.0124816894531250;-0.0161437988281250;-0.0198669433593750;-0.0228271484375000;-0.0272216796875000;-0.0331115722656250;-0.0370178222656250;-0.0401000976562500;-0.0426940917968750;-0.0457153320312500;-0.0485534667968750;-0.0520019531250000;-0.0554809570312500;-0.0570983886718750;-0.0578613281250000;-0.0592041015625000;-0.0590209960937500;-0.0586547851562500;-0.0594177246093750;-0.0607604980468750;-0.0613708496093750;-0.0611572265625000;-0.0611572265625000;-0.0621643066406250;-0.0629272460937500;-0.0640563964843750;-0.0652770996093750;-0.0656433105468750;-0.0655822753906250;-0.0660705566406250;-0.0664062500000000;-0.0669860839843750;-0.0674438476562500;-0.0664062500000000;-0.0654602050781250;-0.0638427734375000;-0.0606079101562500;-0.0564575195312500;-0.0520019531250000;-0.0473327636718750;-0.0430908203125000;-0.0401306152343750;-0.0365905761718750;-0.0314025878906250;-0.0255126953125000;-0.0200500488281250;-0.0167541503906250;-0.0142211914062500;-0.0114746093750000;-0.00894165039062500;-0.00607299804687500;-0.00350952148437500;-0.00192260742187500;0.000396728515625000;0.00332641601562500;0.00643920898437500;0.0105285644531250;0.0141906738281250;0.0150146484375000;0.0149536132812500;0.0155639648437500;0.0171813964843750;0.0181274414062500;0.0184936523437500;0.0192565917968750;0.0196838378906250;0.0206909179687500;0.0210266113281250;0.0205993652343750;0.0195312500000000;0.0194396972656250;0.0202941894531250;0.0212707519531250;0.0227661132812500;0.0243225097656250;0.0264892578125000;0.0286560058593750;0.0297851562500000;0.0298461914062500;0.0288085937500000;0.0286560058593750;0.0292053222656250;0.0297851562500000;0.0305786132812500;0.0309448242187500;0.0315551757812500;0.0307617187500000;0.0280761718750000;0.0253295898437500;0.0233459472656250;0.0198669433593750;0.0155944824218750];
y = [a b*5];
sound(y,Fs);

end
